simulink library "NeuroMuscularLibrary2"  (R2019b)
settings: Solver=ode45  StartTime=0.0  StopTime=10.0  RelTol=1e-3  EnableMultiTasking=on
values from neighbouring files (symbols this model uses):
  c = 0.05    [BodyMechParams.m]
  c_jointstop = 0.3 / (pi/180)    (= 17.1887338539)    [BodyMechParams.m]
  deltaLegAngleThr = 8*pi/180    (= 0.13962634016)    [CMGParams.m]
  DeltaThRef = 2e-3    (= 0.002)    [BodyMechParams.m]
  eref = 0.04    [BodyMechParams.m]
  FmaxGLU = 1500    [BodyMechParams.m]
  footBallToAnkleDist = 0.16    [BodyMechParams.m]
  footBallToCenterDist = footLength/2    (= 0.1)    [BodyMechParams.m]
  footBallToHeelDist = footLength    (= 0.2)    [BodyMechParams.m]
  footCenterToCGDist = 0.14 - footBallToCenterDist    (= 0.04)    [BodyMechParams.m]
  footInertia = 0.005    [BodyMechParams.m]
  footLength = 0.2    [BodyMechParams.m]
  footMass = 1.25    [BodyMechParams.m]
  FT_GLU = 47.6    [BodyMechParams.m]
  g = 9.80665    [BodyMechParams.m]
  groundTheta = [atan(diff(groundZ)./diff(groundX)), 0]    [generateGround.m]
  groundZ = groundZ * stepSize/(largestStep+eps)    [generateGround.m]
  hatHipToCenterDistLen = hatLength/2    (= 0.4)    [BodyMechParams.m]
  hatInertia = 3    [BodyMechParams.m]
  hatLeftHipToCenterDistWidth = .15    (= 0.15)    [BodyMechParams.m]
  hatLength = 0.8    [BodyMechParams.m]
  hatMass = 53.5    [BodyMechParams.m]
  hatThickness = 0.2    [BodyMechParams.m]
  hatWidth = 0.4    [BodyMechParams.m]
  K = 5    [BodyMechParams.m]
  k_gn = k_gn/2    (= 39226.6)    [BodyMechParams.m]
  k_gt = k_gt/2    (= 39226.6)    [BodyMechParams.m]
  k_pressure = hatMass * g / DeltaThRef    (= 262327.8875)    [BodyMechParams.m]
  legAngleSpeedMax = 10    [CMGParams.m]
  loptGAS = 0.05    [BodyMechParams.m]
  loptGLU = 0.11    [BodyMechParams.m]
  loptHAB = 0.09    [BodyMechParams.m]
  loptHAD = 0.10    (= 0.1)    [BodyMechParams.m]
  loptHAM = 0.10    (= 0.1)    [BodyMechParams.m]
  loptHFL = 0.11    [BodyMechParams.m]
  loptSOL = 0.04    [BodyMechParams.m]
  loptTA = 0.06    [BodyMechParams.m]
  loptVAS = 0.08    [BodyMechParams.m]
  lslackGAS = 0.40    (= 0.4)    [BodyMechParams.m]
  lslackGLU = 0.13    [BodyMechParams.m]
  lslackHAB = 0.07    [BodyMechParams.m]
  lslackHAD = 0.18    [BodyMechParams.m]
  lslackHAM = 0.31    [BodyMechParams.m]
  lslackHFL = 0.10    (= 0.1)    [BodyMechParams.m]
  lslackSOL = 0.26    [BodyMechParams.m]
  lslackTA = 0.24    [BodyMechParams.m]
  lslackVAS = 0.23    [BodyMechParams.m]
  mu_slide = 0.8    [BodyMechParams.m]
  mu_stick = 0.9    [BodyMechParams.m]
  N = 1.5    [BodyMechParams.m]    (also in cmaes.m = size(x,1); mergeCompareEnergyCosts.m = {S.name})
  phiKneeUpLimit = 5*pi/180    (= 0.0872664625997)    [BodyMechParams.m]
  phimaxGASa = 20*pi/180    (= 0.349065850399)    [BodyMechParams.m]
  phimaxGASk = 40*pi/180    (= 0.698131700798)    [BodyMechParams.m]
  phimaxHAMk = 0*pi/180    (= 0)    [BodyMechParams.m]
  phimaxSOL = 20*pi/180    (= 0.349065850399)    [BodyMechParams.m]
  phimaxTA = -10*pi/180    (= -0.174532925199)    [BodyMechParams.m]
  phimaxVAS = 15*pi/180    (= 0.261799387799)    [BodyMechParams.m]
  phirefGASa = -10*pi/180    (= -0.174532925199)    [BodyMechParams.m]
  phirefGASk = 15*pi/180    (= 0.261799387799)    [BodyMechParams.m]
  phirefGLU = -30*pi/180    (= -0.523598775598)    [BodyMechParams.m]
  phirefHAB = 10*pi/180    (= 0.174532925199)    [BodyMechParams.m]
  phirefHAD = 15*pi/180    (= 0.261799387799)    [BodyMechParams.m]
  phirefHAMh = -25*pi/180    (= -0.436332312999)    [BodyMechParams.m]
  phirefHAMk = 0*pi/180    (= 0)    [BodyMechParams.m]
  phirefHFL = 0*pi/180    (= 0)    [BodyMechParams.m]
  phirefSOL = -10*pi/180    (= -0.174532925199)    [BodyMechParams.m]
  phirefTA = 20*pi/180    (= 0.349065850399)    [BodyMechParams.m]
  phirefVAS = 55*pi/180    (= 0.959931088597)    [BodyMechParams.m]
  rGASa = 0.05    [BodyMechParams.m]
  rGASk = 0.05    [BodyMechParams.m]
  rGLU = 0.10    (= 0.1)    [BodyMechParams.m]
  rHAB = 0.06    [BodyMechParams.m]
  rHAD = 0.03    [BodyMechParams.m]
  rHAMh = 0.08    [BodyMechParams.m]
  rHAMk = 0.05    [BodyMechParams.m]
  rHFL = 0.10    (= 0.1)    [BodyMechParams.m]
  rhoGASa = 0.7    [BodyMechParams.m]
  rhoGASk = 0.7    [BodyMechParams.m]
  rhoGLU = 0.5    [BodyMechParams.m]
  rhoHAB = 0.7    [BodyMechParams.m]
  rhoHAD = 1    [BodyMechParams.m]
  rhoHAMh = 0.7    [BodyMechParams.m]
  rhoHAMk = 0.7    [BodyMechParams.m]
  rhoHFL = 0.5    [BodyMechParams.m]
  rhoSOL = 0.5    [BodyMechParams.m]
  rhoTA = 0.7    [BodyMechParams.m]
  rhoVAS = 0.7    [BodyMechParams.m]
  RkneeExtendGain = 25000    [CMGParams.m]
  RkneeStopGain = 12000    [CMGParams.m]
  RlegAngleFilter = 100    [CMGParams.m]
  rSOL = 0.05    [BodyMechParams.m]
  rTA = 0.04    [BodyMechParams.m]
  rVAS = 0.06    [BodyMechParams.m]
  s = x(1:N-1,:).^2 + x(2:N,:).^2    [cmaes.m]
  shankAnkleToCenterDist = shankLength/2    (= 0.25)    [BodyMechParams.m]
  shankAnkleToKneeDist = shankLength    (= 0.5)    [BodyMechParams.m]
  shankCenterToCGDist = 0.3 - shankAnkleToCenterDist    (= 0.05)    [BodyMechParams.m]
  shankInertia = 0.05    [BodyMechParams.m]
  shankLength = 0.5    [BodyMechParams.m]
  shankMass = 3.5    [BodyMechParams.m]
  tau = 0.01    [BodyMechParams.m]
  thighCenterToCGDist = 0.3 - thighKneeToCenterDist    (= 0.05)    [BodyMechParams.m]
  thighInertia = 0.15    [BodyMechParams.m]
  thighKneeToCenterDist = thighLength/2    (= 0.25)    [BodyMechParams.m]
  thighKneeToHipDist = thighLength    (= 0.5)    [BodyMechParams.m]
  thighLength = 0.5    [BodyMechParams.m]
  thighMass = 8.5    [BodyMechParams.m]
  v_gn_max = v_gz_max    (= 0.03)    [BodyMechParams.m]
  v_gt_max = v_gz_max    (= 0.03)    [BodyMechParams.m]
  v_max_pressure = 0.5    [BodyMechParams.m]
  vLimit = 0.01    [BodyMechParams.m]
  w = 0.56    [BodyMechParams.m]    (also in MuscleEnergyTest.m = 1.039; cmaes.m = ones(size(x,1)))
  w_max_jointstop = 1 * pi/180    (= 0.0174532925199)    [BodyMechParams.m]
  X = contains(N,'compareEnergyCost') .* ~contains(N,'total') .* ~contains(N,'Total')    [mergeCompareEnergyCosts.m]
undefined symbols (not defined in the file or in its folder): abdHATRef, ankleBackDriveGain, ankleCJointstop, ankleDgain, ankleFilterPID, ankleFilterSEA, ankleGearEff, ankleGearRatio, ankleIgain, ankleInitialAngle, ankleInputMass, ankleIntCoulomb, ankleIntDamping, ankleIntStatic, ankleParallelSpringDamping, ankleParallelSpringOffset, ankleParallelSpringStiffness, anklePgain, anklePlantarLimit, ankleSEADamping, ankleSEAStiffness, ankleTendonMass, ankleWMaxJointstop, dryFrictionDamping, dryFrictionStiffness, dryFrictionVelThresh, footMassp, FourBarL1, FourBarL3, GainCHAB, GainCHAD, GainGAS, GainGLU, GainHAM, GainKneeOverExt, GainSOL, GainSOLTA, GainTA, GainVAS, hipDGain, hipDGainAbd, hipPGain, hipPGainAbd, Kglu, kneeAngleOffset, kneeBackDriveGain, kneeCJointstop, kneeDgain, kneeExtCoulomb, kneeExtDamping, kneeExtendGain, kneeExtStatic, kneeFilterPID, kneeFilterSEA, kneeFlexGain, kneeGearEff, kneeGearRatio, kneeHoldGain1, kneeHoldGain2, kneeIgain ... (+62)
libraries: sm_lib x105, nesl_utility x55, simulink x22, dspswit3 x15, $bdroot x12, simulink_extras x2
(part 2 of 6)

== system NeuroMuscularLibrary2/HAT3D ==
  HAT CG : sm_lib/Frames and Transforms/Reference Frame
  HAT Center to CG : sm_lib/Frames and Transforms/Rigid Transform  TranslationMethod=Cartesian  TranslationStandardOffset=0  TranslationLengthUnit=m  TranslationStandardAxis=+Z  TranslationCartesianOffset=[0, 0, 0]  TranslationROffset=0  TranslationROffsetUnits=m  TranslationZOffset=0  TranslationZOffsetUnits=m  TranslationThetaOffset=0  TranslationThetaOffsetUnits=deg  RotationMethod=None  RotationAngleUnits=deg  RotationStandardAxis=+Z  RotationAngle=0  RotationArbitraryAxis=[0 0 1]  FollAlignAxisA=+X  BaseAlignAxisA=+Y  FollAlignAxisB=+Y  BaseAlignAxisB=+Z  RotationSequenceAxes=FollowerAxes  RotationSequence=XYX  RotationSequenceAngles=[0 0 0]  RotationSequenceAnglesUnits=deg  RotationMatrix=[1 0 0; 0 1 0; 0 0 1]
  HAT Center to Top : sm_lib/Frames and Transforms/Rigid Transform  TranslationMethod=StandardAxis  TranslationStandardOffset=hatLength/2  TranslationLengthUnit=m  TranslationStandardAxis=+Y  TranslationCartesianOffset=[0, 0, 0]  TranslationROffset=0  TranslationROffsetUnits=m  TranslationZOffset=0  TranslationZOffsetUnits=m  TranslationThetaOffset=0  TranslationThetaOffsetUnits=deg  RotationMethod=None  RotationAngleUnits=deg  RotationStandardAxis=+Z  RotationAngle=0  RotationArbitraryAxis=[0 0 1]  FollAlignAxisA=+X  BaseAlignAxisA=+Y  FollAlignAxisB=+Y  BaseAlignAxisB=+Z  RotationSequenceAxes=FollowerAxes  RotationSequence=XYX  RotationSequenceAngles=[0 0 0]  RotationSequenceAnglesUnits=deg  RotationMatrix=[1 0 0; 0 1 0; 0 0 1]
  Hip Solid : sm_lib/Body Elements/Brick Solid  GraphicAmbientColor=[0.15 0.15 0.15 1.0]  BasedOnType=Density  BrickDimensions=[hatThickness, hatLength, hatWidth]  BrickDimensionUnits=m  CenterOfMass=[0, 0, 0]  CenterOfMassUnits=m  GraphicDiffuseColor=[0.5 0.5 0.5]  Density=1000  DensityUnits=kg/(m^3)  DoExposeReferenceFrame=on  GraphicEmissiveColor=[0.0 0.0 0.0 1.0]  ExportEntireGeometry=off  SerializedFrames=<Frames/>  MarkerShape=Sphere  MarkerSize=10  GraphicType=FromGeometry  InertiaType=Custom  Mass=hatMass  MassUnits=kg  MomentsOfInertia=[0 0 hatInertia]  MomentsOfInertiaUnits=kg*m^2  GraphicOpacity=1.0  ProductsOfInertia=[0 0 0]  ProductsOfInertiaUnits=kg*m^2  GraphicShininess=75  GraphicSpecularColor=[0.5 0.5 0.5 1.0]  GraphicVisPropType=SimpleVisualProperties
  Left Hip to Center : sm_lib/Frames and Transforms/Rigid Transform  TranslationMethod=Cartesian  TranslationStandardOffset=0  TranslationLengthUnit=m  TranslationStandardAxis=+Z  TranslationCartesianOffset=[0, hatHipToCenterDistLen, hatLeftHipToCenterDistWidth]  TranslationROffset=0  TranslationROffsetUnits=m  TranslationZOffset=0  TranslationZOffsetUnits=m  TranslationThetaOffset=0  TranslationThetaOffsetUnits=deg  RotationMethod=None  RotationAngleUnits=deg  RotationStandardAxis=+Z  RotationAngle=0  RotationArbitraryAxis=[0 0 1]  FollAlignAxisA=+X  BaseAlignAxisA=+Y  FollAlignAxisB=+Y  BaseAlignAxisB=+Z  RotationSequenceAxes=FollowerAxes  RotationSequence=XYX  RotationSequenceAngles=[0 0 0]  RotationSequenceAnglesUnits=deg  RotationMatrix=[1 0 0; 0 1 0; 0 0 1]
  Left Hip to Right Hip : sm_lib/Frames and Transforms/Rigid Transform  TranslationMethod=Cartesian  TranslationStandardOffset=0  TranslationLengthUnit=m  TranslationStandardAxis=+Z  TranslationCartesianOffset=[0 0 2*hatLeftHipToCenterDistWidth]  TranslationROffset=0  TranslationROffsetUnits=m  TranslationZOffset=0  TranslationZOffsetUnits=m  TranslationThetaOffset=0  TranslationThetaOffsetUnits=deg  RotationMethod=None  RotationAngleUnits=deg  RotationStandardAxis=+Z  RotationAngle=0  RotationArbitraryAxis=[0 0 1]  FollAlignAxisA=+X  BaseAlignAxisA=+Y  FollAlignAxisB=+Y  BaseAlignAxisB=+Z  RotationSequenceAxes=FollowerAxes  RotationSequence=XYX  RotationSequenceAngles=[0 0 0]  RotationSequenceAnglesUnits=deg  RotationMatrix=[1 0 0; 0 1 0; 0 0 1]
  Mux : Mux  Inputs=2
  Mux1 : Mux  Inputs=2
  PS-Simulink Converter{,1..3} (4 alike) : nesl_utility/PS-Simulink Converter  PhysicalDomain=network_engine_domain  SubClassName=ps_output  LeftPortType=input  RightPortType=output  PseudoPeriodic=off  Frequencies=[]  Unit=1  AffineConversion=off
  To: X-forward Y-Lateral Z-up : sm_lib/Frames and Transforms/Rigid Transform  TranslationMethod=None  TranslationStandardOffset=0  TranslationLengthUnit=m  TranslationStandardAxis=+Z  TranslationCartesianOffset=[0, hatHipToCenterDistLen, -hatLeftHipToCenterDistWidth]  TranslationROffset=0  TranslationROffsetUnits=m  TranslationZOffset=0  TranslationZOffsetUnits=m  TranslationThetaOffset=0  TranslationThetaOffsetUnits=deg  RotationMethod=AlignedAxes  RotationAngleUnits=deg  RotationStandardAxis=+Z  RotationAngle=0  RotationArbitraryAxis=[0 0 1]  FollAlignAxisA=+X  BaseAlignAxisA=+Z  FollAlignAxisB=+Z  BaseAlignAxisB=+Y  RotationSequenceAxes=FollowerAxes  RotationSequence=XYX  RotationSequenceAngles=[0 0 0]  RotationSequenceAnglesUnits=deg  RotationMatrix=[1 0 0; 0 1 0; 0 0 1]
  To: Z-forward X-Lateral Y-up : sm_lib/Frames and Transforms/Rigid Transform  TranslationMethod=None  TranslationStandardOffset=0  TranslationLengthUnit=m  TranslationStandardAxis=+Z  TranslationCartesianOffset=[0, hatHipToCenterDistLen, -hatLeftHipToCenterDistWidth]  TranslationROffset=0  TranslationROffsetUnits=m  TranslationZOffset=0  TranslationZOffsetUnits=m  TranslationThetaOffset=0  TranslationThetaOffsetUnits=deg  RotationMethod=AlignedAxes  RotationAngleUnits=deg  RotationStandardAxis=+Z  RotationAngle=0  RotationArbitraryAxis=[0 0 1]  FollAlignAxisA=+Y  BaseAlignAxisA=+Y  FollAlignAxisB=+Z  BaseAlignAxisB=+X  RotationSequenceAxes=FollowerAxes  RotationSequence=XYX  RotationSequenceAngles=[0 0 0]  RotationSequenceAnglesUnits=deg  RotationMatrix=[1 0 0; 0 1 0; 0 0 1]
  Transform Sensor : sm_lib/Frames and Transforms/Transform Sensor  MeasurementFrame=World  SenseAngle=on  SenseAxis=off  SenseAngle1=off  SenseAngle2=off  SenseAngle3=off  SenseQ=off  SenseR=off  SenseOmegaX=off  SenseOmegaY=on  SenseOmegaZ=off  SenseOmega1=off  SenseOmega2=off  SenseOmega3=off  SenseQDot=off  SenseRDot=off  SenseAlphaX=off  SenseAlphaY=off  SenseAlphaZ=off  SenseAlpha1=off  SenseAlpha2=off  SenseAlpha3=off  SenseQDDot=off  SenseRDDot=off  SenseX=off  SenseY=off  SenseZ=off  SenseRad=off  SenseAzim=off  SenseDist=off  SenseInc=off  SenseXDot=off  SenseYDot=off  SenseZDot=off  SenseRadDot=off  SenseAzimDot=off  SenseDistDot=off  SenseIncDot=off  SenseXDDot=off  SenseYDDot=off  SenseZDDot=off  SenseRadDDot=off  SenseAzimDDot=off  SenseDistDDot=off  SenseIncDDot=off
  Transform Sensor : sm_lib/Frames and Transforms/Transform Sensor  MeasurementFrame=World  SenseAngle=on  SenseAxis=off  SenseAngle1=off  SenseAngle2=off  SenseAngle3=off  SenseQ=off  SenseR=off  SenseOmegaX=off  SenseOmegaY=on  SenseOmegaZ=off  SenseOmega1=off  SenseOmega2=off  SenseOmega3=off  SenseQDot=off  SenseRDot=off  SenseAlphaX=off  SenseAlphaY=off  SenseAlphaZ=off  SenseAlpha1=off  SenseAlpha2=off  SenseAlpha3=off  SenseQDDot=off  SenseRDDot=off  SenseX=off  SenseY=off  SenseZ=off  SenseRad=off  SenseAzim=off  SenseDist=off  SenseInc=off  SenseXDot=off  SenseYDot=off  SenseZDot=off  SenseRadDot=off  SenseAzimDot=off  SenseDistDot=off  SenseIncDot=off  SenseXDDot=off  SenseYDDot=off  SenseZDDot=off  SenseRadDDot=off  SenseAzimDDot=off  SenseDistDDot=off  SenseIncDDot=off
  World Frame : sm_lib/Frames and Transforms/World Frame
  Left Hip : PMIOPort  Side=Left
  Right Hip : PMIOPort  Port=2  Side=Left
  HATTop : PMIOPort  Port=3  Side=Right
  CG : PMIOPort  Port=4  Side=Right
  phiANDdphiHAT : Outport
  phiANDdphiHATAbd : Outport  Port=2
  wires:
  PS-Simulink Converter2/1 -> Mux1/1
  Mux1/1 -> phiANDdphiHATAbd/1
  PS-Simulink Converter3/1 -> Mux1/2
  PS-Simulink Converter/1 -> Mux/1
  PS-Simulink Converter1/1 -> Mux/2
  Mux/1 -> phiANDdphiHAT/1
  connections:
  Transform Sensor/RConn2 -- PS-Simulink Converter2/LConn1
  Transform Sensor/RConn3 -- PS-Simulink Converter3/LConn1
  To: Z-forward X-Lateral Y-up/RConn1 -- Transform Sensor/RConn1 -- To: X-forward Y-Lateral Z-up/LConn1
  Left Hip/RConn1 -- To: Z-forward X-Lateral Y-up/LConn1 -- Left Hip to Center/LConn1 -- Left Hip to Right Hip/LConn1
  Left Hip to Center/RConn1 -- HAT Center to CG/LConn1 -- Hip Solid/RConn1 -- HAT Center to Top/LConn1
  Right Hip/RConn1 -- Left Hip to Right Hip/RConn1
  World Frame/RConn1 -- Transform Sensor/LConn1
  PS-Simulink Converter/LConn1 -- Transform Sensor/RConn2
  Transform Sensor/RConn3 -- PS-Simulink Converter1/LConn1
  To: X-forward Y-Lateral Z-up/RConn1 -- Transform Sensor/RConn1
  HAT CG/RConn1 -- HAT Center to CG/RConn1 -- CG/RConn1
  HATTop/RConn1 -- HAT Center to Top/RConn1

== system NeuroMuscularLibrary2/HFL Link ==
  note: HFL Attachment
  hip angle [rad] : Inport
  Constant : Constant  Value=lslackHFL+loptHFL
  Constant1 : Constant  Value=rHFL
  Constant2 : Constant  Value=phirefHFL
  Gain2 : Gain  Gain=rhoHFL
  Product : Product  RndMeth=Zero
  Sum2 : Sum  Inputs=|+-
  Sum5 : Sum  Inputs=|++
  lmtu [m] : Outport
  lever [m] : Outport  Port=2
  wires:
  Constant/1 -> Sum5/1
  Sum5/1 -> lmtu [m]/1
  Product/1 -> Gain2/1
  hip angle [rad]/1 -> Sum2/1
  Constant2/1 -> Sum2/2
  Sum2/1 -> Product/1
  Constant1/1 -> Product/2, lever [m]/1
  Gain2/1 -> Sum5/2

== system NeuroMuscularLibrary2/Hard Stops ==
  Ideal Torques : Inport
  Muscle Torques : Inport  Port=2
  phiANDdphiHip : Inport  Port=3
  phiANDdphiKnee : Inport  Port=4
  phiANDdphiAnkle : Inport  Port=5
  Add : Sum  Inputs=+++
  Ankle Joint Limit : $bdroot/Overextension//Overflexion Joint Limit  phiUpLimit=phiAnkleUpLimit  phiLowLimit=phiAnkleLowLimit
  Demux : Demux  Outputs=2
  Demux1 : Demux  Outputs=2
  Demux2 : Demux  Outputs=2
  Hip Overextension Joint Limit : $bdroot/Overextension Joint Limit  phiUpLimit=phiHipUpLimit  ext=1
  Knee Overextension Joint Limit : $bdroot/Overextension Joint Limit  phiUpLimit=phiKneeUpLimit  ext=-1
  Mux : Mux  Inputs=3
  Over Extended Knee? : simulink/Logic and Bit Operations/Compare To Constant  relop=<  const=-5*pi/180  OutDataTypeStr=boolean
  Product1 : Product
  Net Torque : Outport
  Hip Stop Torque : Outport  Port=2
  Knee Stop Torque : Outport  Port=3
  Ankle Stop Torque : Outport  Port=4
  wires:
  Ideal Torques/1 -> Add/1
  Add/1 -> Net Torque/1
  phiANDdphiAnkle/1 -> Demux2/1
  phiANDdphiHip/1 -> Demux1/1
  Hip Overextension Joint Limit/1 -> Mux/1, Hip Stop Torque/1
  phiANDdphiKnee/1 -> Demux/1
  Demux2/2 -> Ankle Joint Limit/2
  Demux2/1 -> Ankle Joint Limit/1
  Demux1/2 -> Hip Overextension Joint Limit/2
  Demux1/1 -> Hip Overextension Joint Limit/1
  Demux/1 -> Knee Overextension Joint Limit/1, Over Extended Knee?/1
  Demux/2 -> Knee Overextension Joint Limit/2
  Over Extended Knee?/1 -> Product1/2
  Ankle Joint Limit/1 -> Mux/3, Ankle Stop Torque/1
  Mux/1 -> Add/3
  Muscle Torques/1 -> Add/2
  Knee Overextension Joint Limit/1 -> Product1/1, Mux/2
  Product1/1 -> Knee Stop Torque/1

== system NeuroMuscularLibrary2/Hard Stops 3D ==
  Ideal Torques : Inport
  Muscle Torques : Inport  Port=2
  phiANDdphiHip : Inport  Port=3
  phiANDdphiKnee : Inport  Port=4
  phiANDdphiAnkle : Inport  Port=5
  phiANDdphiHipAbd : Inport  Port=6
  Add : Sum  Inputs=+++
  Ankle Joint Limit : $bdroot/Overextension//Overflexion Joint Limit  phiUpLimit=phiAnkleUpLimit  phiLowLimit=phiAnkleLowLimit
  Demux{,1..3} (4 alike) : Demux  Outputs=2
  Hip Abduction Joint Limit : $bdroot/Overextension//Overflexion Joint Limit  phiUpLimit=phiHipAbdUpLimit  phiLowLimit=phiHipAbdLowLimit
  Hip Overextension Joint Limit : $bdroot/Overextension Joint Limit  phiUpLimit=phiHipUpLimit  ext=1
  Knee Overextension Joint Limit : $bdroot/Overextension Joint Limit  phiUpLimit=phiKneeUpLimit  ext=-1
  Mux : Mux
  Over Extended Knee? : simulink/Logic and Bit Operations/Compare To Constant  relop=<  const=-5*pi/180  OutDataTypeStr=boolean
  Product1 : Product
  Net Torque : Outport
  Hip Stop Torque : Outport  Port=2
  Knee Stop Torque : Outport  Port=3
  Ankle Stop Torque : Outport  Port=4
  Hip Abd Stop Torque : Outport  Port=5
  wires:
  Product1/1 -> Knee Stop Torque/1
  Knee Overextension Joint Limit/1 -> Mux/2, Product1/1
  Muscle Torques/1 -> Add/2
  Mux/1 -> Add/3
  Ankle Joint Limit/1 -> Ankle Stop Torque/1, Mux/3
  Over Extended Knee?/1 -> Product1/2
  Demux/2 -> Knee Overextension Joint Limit/2
  Demux/1 -> Over Extended Knee?/1, Knee Overextension Joint Limit/1
  Demux1/1 -> Hip Overextension Joint Limit/1
  Demux1/2 -> Hip Overextension Joint Limit/2
  Demux2/1 -> Ankle Joint Limit/1
  Demux2/2 -> Ankle Joint Limit/2
  phiANDdphiKnee/1 -> Demux/1
  Hip Overextension Joint Limit/1 -> Hip Stop Torque/1, Mux/1
  phiANDdphiHip/1 -> Demux1/1
  phiANDdphiAnkle/1 -> Demux2/1
  Add/1 -> Net Torque/1
  Ideal Torques/1 -> Add/1
  phiANDdphiHipAbd/1 -> Demux3/1
  Demux3/1 -> Hip Abduction Joint Limit/1
  Demux3/2 -> Hip Abduction Joint Limit/2
  Hip Abduction Joint Limit/1 -> Hip Abd Stop Torque/1, Mux/4

== system NeuroMuscularLibrary2/Hill Muscle ==
  note: Muscle-Tendon Dynamics
  note: Excitation Contraction Coupling
  STIM : Inport
  lmtc [m] : Inport  Port=2
  1 : Product  Inputs=**  SaturateOnIntegerOverflow=on  InputSameDT=on  OutDataTypeStr=Inherit: Same as first input
  1/lslack : Gain  Gain=1/lslack  SaturateOnIntegerOverflow=on  OutDataTypeStr=Inherit: Same as input  ParamDataTypeStr=Inherit: Same as input
  BE force-length relation : Subsystem
  CE force-length relation : Subsystem
  CE inverse force-velocity relation : Subsystem
  Constant : Constant  Value=lslack
  ECC TransferFcn : simulink_extras/Additional Linear/Transfer Fcn (with initial outputs)  N=[1]  D="[tau  1]"  Y0=preA  U0=0
      settings: AttributesFormatString=pre-activation: %<Y0>
  Fmax : Gain  Gain=Fmax  SaturateOnIntegerOverflow=on  OutDataTypeStr=Inherit: Same as input  ParamDataTypeStr=Inherit: Same as input
  Fv = Fse / (A*Fce) : Product  Inputs=*/  SaturateOnIntegerOverflow=on  InputSameDT=on  OutDataTypeStr=Inherit: Same as first input
  Integrator : Integrator  InitialConditionSource=external  LowerSaturationLimit=0.05
  PE force-length relation : Subsystem
  SE force-length relation : Subsystem
  Sum : Sum  Inputs=|+-  SaturateOnIntegerOverflow=on  InputSameDT=on  OutDataTypeStr=Inherit: Same as first input
  Sum2 : Sum  Inputs=|-+  SaturateOnIntegerOverflow=on  InputSameDT=on  OutDataTypeStr=Inherit: Same as first input
  Sum3 : Sum  SaturateOnIntegerOverflow=on  InputSameDT=on  OutDataTypeStr=Inherit: Same as first input
  Sum4 : Sum  SaturateOnIntegerOverflow=on  InputSameDT=on  OutDataTypeStr=Inherit: Same as first input
  lce/lopt : Gain  Gain=1/lopt  SaturateOnIntegerOverflow=on  OutDataTypeStr=Inherit: Same as input  ParamDataTypeStr=Inherit: Same as input
  vmax*lopt : Gain  Gain=vmax*lopt  SaturateOnIntegerOverflow=on  OutDataTypeStr=Inherit: Same as input  ParamDataTypeStr=Inherit: Same as input
  Fmtc : Outport  InitialOutput=0
  Lce : Outport  Port=2  InitialOutput=0
  Vce : Outport  Port=3  InitialOutput=0
  Lse : Outport  Port=4  InitialOutput=0
  A : Outport  Port=5  InitialOutput=0
  wires:
  Integrator/1 -> Sum/2, lce/lopt/1, Lce/1  "lce"
  Sum/1 -> 1/lslack/1, Lse/1  "lse"
  lce/lopt/1 -> CE force-length relation/1(lce [lopt]), BE force-length relation/1(lce [lopt]), PE force-length relation/1(lce [lopt])
  Fv = Fse / (A*Fce)/1 -> CE inverse force-velocity relation/1(Fv[Fmax])  "fv"
  vmax*lopt/1 -> Integrator/1, Vce/1  "vce"
  lmtc [m]/1 -> Sum2/2, Sum/1  "lmtc"
  Fmax/1 -> Fmtc/1  "Fmtc"
  1/lslack/1 -> SE force-length relation/1(lse [lslack])
  SE force-length relation/1(fse [Fmax]) -> Fmax/1, Sum4/1
  Sum2/1 -> Integrator/2
  Constant/1 -> Sum2/1
  CE force-length relation/1(fce [Fmax]) -> 1/1
  Sum4/1 -> Fv = Fse / (A*Fce)/1
  PE force-length relation/1(fpe [Fmax]) -> Sum3/1
  1/1 -> Sum3/2
  BE force-length relation/1(fbe [Fmax]) -> Sum4/2
  Sum3/1 -> Fv = Fse / (A*Fce)/2
  CE inverse force-velocity relation/1(v[vmax]) -> vmax*lopt/1
  STIM/1 -> ECC TransferFcn/1
  ECC TransferFcn/1 -> A/1, 1/2

== system NeuroMuscularLibrary2/Leg Angle//Length ==
  Constant : Constant  Value=pi
  Demux : Demux  Outputs=2
  Mux : Mux  Inputs=3
  Mux1 : Mux  Inputs=3
  PS-Simulink Converter{,1..6} (7 alike) : nesl_utility/PS-Simulink Converter  PhysicalDomain=network_engine_domain  SubClassName=ps_output  LeftPortType=input  RightPortType=output  PseudoPeriodic=off  Frequencies=[]  Unit=m  AffineConversion=off
  Position Sensor : sm_lib/Frames and Transforms/Transform Sensor  MeasurementFrame=World  SenseAngle=off  SenseAxis=off  SenseAngle1=off  SenseAngle2=off  SenseAngle3=off  SenseQ=off  SenseR=off  SenseOmegaX=off  SenseOmegaY=off  SenseOmegaZ=off  SenseOmega1=off  SenseOmega2=off  SenseOmega3=off  SenseQDot=off  SenseRDot=off  SenseAlphaX=off  SenseAlphaY=off  SenseAlphaZ=off  SenseAlpha1=off  SenseAlpha2=off  SenseAlpha3=off  SenseQDDot=off  SenseRDDot=off  SenseX=on  SenseY=on  SenseZ=on  SenseRad=off  SenseAzim=off  SenseDist=off  SenseInc=off  SenseXDot=off  SenseYDot=off  SenseZDot=off  SenseRadDot=off  SenseAzimDot=off  SenseDistDot=off  SenseIncDot=off  SenseXDDot=off  SenseYDDot=off  SenseZDDot=off  SenseRadDDot=off  SenseAzimDDot=off  SenseDistDDot=off  SenseIncDDot=off
  Position Sensor1 : sm_lib/Frames and Transforms/Transform Sensor  MeasurementFrame=World  SenseAngle=off  SenseAxis=off  SenseAngle1=off  SenseAngle2=off  SenseAngle3=off  SenseQ=off  SenseR=off  SenseOmegaX=off  SenseOmegaY=off  SenseOmegaZ=off  SenseOmega1=off  SenseOmega2=off  SenseOmega3=off  SenseQDot=off  SenseRDot=off  SenseAlphaX=off  SenseAlphaY=off  SenseAlphaZ=off  SenseAlpha1=off  SenseAlpha2=off  SenseAlpha3=off  SenseQDDot=off  SenseRDDot=off  SenseX=on  SenseY=on  SenseZ=on  SenseRad=off  SenseAzim=off  SenseDist=off  SenseInc=off  SenseXDot=off  SenseYDot=off  SenseZDot=off  SenseRadDot=off  SenseAzimDot=off  SenseDistDot=off  SenseIncDot=off  SenseXDDot=off  SenseYDDot=off  SenseZDDot=off  SenseRadDDot=off  SenseAzimDDot=off  SenseDistDDot=off  SenseIncDDot=off
  Selector : Selector  InputPortWidth=3  IndexOptions=Index vector (dialog)  Indices=[3 1]  OutputSizes=1
  Subtract : Sum  Inputs=+-
  Sum : Sum  Inputs=|-+
  Transform Sensor : sm_lib/Frames and Transforms/Transform Sensor  MeasurementFrame=World  SenseAngle=off  SenseAxis=off  SenseAngle1=off  SenseAngle2=off  SenseAngle3=off  SenseQ=off  SenseR=off  SenseOmegaX=off  SenseOmegaY=off  SenseOmegaZ=off  SenseOmega1=off  SenseOmega2=off  SenseOmega3=off  SenseQDot=off  SenseRDot=off  SenseAlphaX=off  SenseAlphaY=off  SenseAlphaZ=off  SenseAlpha1=off  SenseAlpha2=off  SenseAlpha3=off  SenseQDDot=off  SenseRDDot=off  SenseX=off  SenseY=off  SenseZ=off  SenseRad=off  SenseAzim=off  SenseDist=on  SenseInc=off  SenseXDot=off  SenseYDot=off  SenseZDot=off  SenseRadDot=off  SenseAzimDot=off  SenseDistDot=off  SenseIncDot=off  SenseXDDot=off  SenseYDDot=off  SenseZDDot=off  SenseRadDDot=off  SenseAzimDDot=off  SenseDistDDot=off  SenseIncDDot=off
  Trigonometric Function : Trigonometry  Operator=atan2  OutputSignalType=real
  World Frame : sm_lib/Frames and Transforms/World Frame
  Hip : PMIOPort  Side=Left
  Ankle : PMIOPort  Port=2  Side=Left
  Leg Angle : Outport
  Leg Length : Outport  Port=2
  wires:
  PS-Simulink Converter6/1 -> Leg Length/1
  PS-Simulink Converter2/1 -> Mux/3
  PS-Simulink Converter/1 -> Mux/1
  PS-Simulink Converter1/1 -> Mux/2
  PS-Simulink Converter5/1 -> Mux1/3
  PS-Simulink Converter3/1 -> Mux1/1
  PS-Simulink Converter4/1 -> Mux1/2
  Mux/1 -> Subtract/1
  Mux1/1 -> Subtract/2
  Trigonometric Function/1 -> Sum/1
  Sum/1 -> Leg Angle/1  "Saggital leg angle"
  Constant/1 -> Sum/2
  Subtract/1 -> Selector/1
  Selector/1 -> Demux/1
  Demux/1 -> Trigonometric Function/1
  Demux/2 -> Trigonometric Function/2
  connections:
  PS-Simulink Converter6/LConn1 -- Transform Sensor/RConn2
  PS-Simulink Converter2/LConn1 -- Position Sensor/RConn4
  PS-Simulink Converter/LConn1 -- Position Sensor/RConn2
  Transform Sensor/RConn1 -- Hip/RConn1 -- Position Sensor/RConn1
  PS-Simulink Converter1/LConn1 -- Position Sensor/RConn3
  World Frame/RConn1 -- Position Sensor/LConn1 -- Position Sensor1/LConn1
  PS-Simulink Converter4/LConn1 -- Position Sensor1/RConn3
  PS-Simulink Converter5/LConn1 -- Position Sensor1/RConn4
  PS-Simulink Converter3/LConn1 -- Position Sensor1/RConn2
  Transform Sensor/LConn1 -- Ankle/RConn1 -- Position Sensor1/RConn1

== system NeuroMuscularLibrary2/Leg Angle//Length3D ==
  Constant : Constant  Value=pi
  Constant1 : Constant  Value=0
  Demux : Demux  Outputs=2
  Demux1 : Demux  Outputs=2
  Mux : Mux  Inputs=3
  Mux1 : Mux  Inputs=3
  Mux2 : Mux  Inputs=2
  PS-Simulink Converter{,1..6} (7 alike) : nesl_utility/PS-Simulink Converter  PhysicalDomain=network_engine_domain  SubClassName=ps_output  LeftPortType=input  RightPortType=output  PseudoPeriodic=off  Frequencies=[]  Unit=m  AffineConversion=off
  Position Sensor : sm_lib/Frames and Transforms/Transform Sensor  MeasurementFrame=World  SenseAngle=off  SenseAxis=off  SenseAngle1=off  SenseAngle2=off  SenseAngle3=off  SenseQ=off  SenseR=off  SenseOmegaX=off  SenseOmegaY=off  SenseOmegaZ=off  SenseOmega1=off  SenseOmega2=off  SenseOmega3=off  SenseQDot=off  SenseRDot=off  SenseAlphaX=off  SenseAlphaY=off  SenseAlphaZ=off  SenseAlpha1=off  SenseAlpha2=off  SenseAlpha3=off  SenseQDDot=off  SenseRDDot=off  SenseX=on  SenseY=on  SenseZ=on  SenseRad=off  SenseAzim=off  SenseDist=off  SenseInc=off  SenseXDot=off  SenseYDot=off  SenseZDot=off  SenseRadDot=off  SenseAzimDot=off  SenseDistDot=off  SenseIncDot=off  SenseXDDot=off  SenseYDDot=off  SenseZDDot=off  SenseRadDDot=off  SenseAzimDDot=off  SenseDistDDot=off  SenseIncDDot=off
  Position Sensor1 : sm_lib/Frames and Transforms/Transform Sensor  MeasurementFrame=World  SenseAngle=off  SenseAxis=off  SenseAngle1=off  SenseAngle2=off  SenseAngle3=off  SenseQ=off  SenseR=off  SenseOmegaX=off  SenseOmegaY=off  SenseOmegaZ=off  SenseOmega1=off  SenseOmega2=off  SenseOmega3=off  SenseQDot=off  SenseRDot=off  SenseAlphaX=off  SenseAlphaY=off  SenseAlphaZ=off  SenseAlpha1=off  SenseAlpha2=off  SenseAlpha3=off  SenseQDDot=off  SenseRDDot=off  SenseX=on  SenseY=on  SenseZ=on  SenseRad=off  SenseAzim=off  SenseDist=off  SenseInc=off  SenseXDot=off  SenseYDot=off  SenseZDot=off  SenseRadDot=off  SenseAzimDot=off  SenseDistDot=off  SenseIncDot=off  SenseXDDot=off  SenseYDDot=off  SenseZDDot=off  SenseRadDDot=off  SenseAzimDDot=off  SenseDistDDot=off  SenseIncDDot=off
  Selector : Selector  InputPortWidth=3  IndexOptions=Index vector (dialog)  Indices=[3 1]  OutputSizes=1
  Selector1 : Selector  InputPortWidth=3  IndexOptions=Index vector (dialog)  Indices=[3 2]  OutputSizes=1
  Subtract : Sum  Inputs=+-
  Sum : Sum  Inputs=|-+
  Sum1 : Sum  Inputs=|++
  Transform Sensor : sm_lib/Frames and Transforms/Transform Sensor  MeasurementFrame=World  SenseAngle=off  SenseAxis=off  SenseAngle1=off  SenseAngle2=off  SenseAngle3=off  SenseQ=off  SenseR=off  SenseOmegaX=off  SenseOmegaY=off  SenseOmegaZ=off  SenseOmega1=off  SenseOmega2=off  SenseOmega3=off  SenseQDot=off  SenseRDot=off  SenseAlphaX=off  SenseAlphaY=off  SenseAlphaZ=off  SenseAlpha1=off  SenseAlpha2=off  SenseAlpha3=off  SenseQDDot=off  SenseRDDot=off  SenseX=off  SenseY=off  SenseZ=off  SenseRad=off  SenseAzim=off  SenseDist=on  SenseInc=off  SenseXDot=off  SenseYDot=off  SenseZDot=off  SenseRadDot=off  SenseAzimDot=off  SenseDistDot=off  SenseIncDot=off  SenseXDDot=off  SenseYDDot=off  SenseZDDot=off  SenseRadDDot=off  SenseAzimDDot=off  SenseDistDDot=off  SenseIncDDot=off
  Trigonometric Function : Trigonometry  Operator=atan2  OutputSignalType=real
  Trigonometric Function1 : Trigonometry  Operator=atan2  OutputSignalType=real
  World Frame : sm_lib/Frames and Transforms/World Frame
  Hip : PMIOPort  Side=Left
  Ankle : PMIOPort  Port=2  Side=Left
  Leg Angle : Outport
  Leg Length : Outport  Port=2
  wires:
  Sum1/1 -> Mux2/2  "Coronal leg angle"
  Trigonometric Function1/1 -> Sum1/1
  Constant1/1 -> Sum1/2
  Demux1/2 -> Trigonometric Function1/2
  Selector1/1 -> Demux1/1
  Demux1/1 -> Trigonometric Function1/1
  Mux2/1 -> Leg Angle/1
  Demux/2 -> Trigonometric Function/2
  Demux/1 -> Trigonometric Function/1
  Selector/1 -> Demux/1
  Subtract/1 -> Selector/1, Selector1/1
  Constant/1 -> Sum/2
  Sum/1 -> Mux2/1  "Saggital leg angle"
  Trigonometric Function/1 -> Sum/1
  Mux1/1 -> Subtract/2
  Mux/1 -> Subtract/1
  PS-Simulink Converter4/1 -> Mux1/2
  PS-Simulink Converter3/1 -> Mux1/1
  PS-Simulink Converter5/1 -> Mux1/3
  PS-Simulink Converter1/1 -> Mux/2
  PS-Simulink Converter/1 -> Mux/1
  PS-Simulink Converter2/1 -> Mux/3
  PS-Simulink Converter6/1 -> Leg Length/1
  connections:
  Position Sensor1/RConn1 -- Ankle/RConn1 -- Transform Sensor/LConn1
  PS-Simulink Converter3/LConn1 -- Position Sensor1/RConn2
  PS-Simulink Converter5/LConn1 -- Position Sensor1/RConn4
  PS-Simulink Converter4/LConn1 -- Position Sensor1/RConn3
  Position Sensor1/LConn1 -- Position Sensor/LConn1 -- World Frame/RConn1
  PS-Simulink Converter1/LConn1 -- Position Sensor/RConn3
  Position Sensor/RConn1 -- Hip/RConn1 -- Transform Sensor/RConn1
  PS-Simulink Converter/LConn1 -- Position Sensor/RConn2
  PS-Simulink Converter2/LConn1 -- Position Sensor/RConn4
  PS-Simulink Converter6/LConn1 -- Transform Sensor/RConn2

== system NeuroMuscularLibrary2/Lower Thigh ==
  Knee Solid : sm_lib/Body Elements/Cylindrical Solid  GraphicAmbientColor=[0.15 0.15 0.15 1.0]  BasedOnType=Density  CenterOfMass=[0 0 thighCenterToCGDist*ThPos]  CenterOfMassUnits=m  GraphicDiffuseColor=[0.5 0.5 0.5]  CylinderLength=thighLength*ThPos  CylinderLengthUnits=m  CylinderRadius=.075  CylinderRadiusUnits=m  Density=1000  DensityUnits=kg/(m^3)  DoExposeReferenceFrame=on  GraphicEmissiveColor=[0.0 0.0 0.0 1.0]  ExportEntireGeometry=off  SerializedFrames=<Frames/>  MarkerShape=Sphere  MarkerSize=10  GraphicType=FromGeometry  InertiaType=Custom  Mass=thighMass*ThPos  MassUnits=kg  MomentsOfInertia=[thighInertia*(ThPos)^3 0 0]  MomentsOfInertiaUnits=kg*m^2  GraphicOpacity=1.0  ProductsOfInertia=[0 0 0]  ProductsOfInertiaUnits=kg*m^2  GraphicShininess=75  GraphicSpecularColor=[0.5 0.5 0.5 1.0]  GraphicVisPropType=SimpleVisualProperties
  Knee to Center : sm_lib/Frames and Transforms/Rigid Transform  TranslationMethod=Cartesian  TranslationStandardOffset=0  TranslationLengthUnit=m  TranslationStandardAxis=+Z  TranslationCartesianOffset=[0 thighKneeToCenterDist*ThPos 0]  TranslationROffset=0  TranslationROffsetUnits=m  TranslationZOffset=0  TranslationZOffsetUnits=m  TranslationThetaOffset=0  TranslationThetaOffsetUnits=deg  RotationMethod=AlignedAxes  RotationAngleUnits=deg  RotationStandardAxis=+Z  RotationAngle=0  RotationArbitraryAxis=[0 0 1]  FollAlignAxisA=+Z  BaseAlignAxisA=+Y  FollAlignAxisB=+X  BaseAlignAxisB=+X  RotationSequenceAxes=FollowerAxes  RotationSequence=XYX  RotationSequenceAngles=[0 0 0]  RotationSequenceAnglesUnits=deg  RotationMatrix=[1 0 0; 0 1 0; 0 0 1]
  Knee to Sensor Sheet : sm_lib/Frames and Transforms/Rigid Transform  TranslationMethod=Cartesian  TranslationStandardOffset=0  TranslationLengthUnit=m  TranslationStandardAxis=+Z  TranslationCartesianOffset=[0 thighKneeToHipDist*ThPos 0]  TranslationROffset=0  TranslationROffsetUnits=m  TranslationZOffset=0  TranslationZOffsetUnits=m  TranslationThetaOffset=0  TranslationThetaOffsetUnits=deg  RotationMethod=None  RotationAngleUnits=deg  RotationStandardAxis=+Z  RotationAngle=0  RotationArbitraryAxis=[0 0 1]  FollAlignAxisA=+Z  BaseAlignAxisA=+X  FollAlignAxisB=+Y  BaseAlignAxisB=+Y  RotationSequenceAxes=FollowerAxes  RotationSequence=XYX  RotationSequenceAngles=[0 0 0]  RotationSequenceAnglesUnits=deg  RotationMatrix=[1 0 0; 0 1 0; 0 0 1]
  Thigh CG : sm_lib/Frames and Transforms/Reference Frame
  Thigh Center to CG : sm_lib/Frames and Transforms/Rigid Transform  TranslationMethod=Cartesian  TranslationStandardOffset=0  TranslationLengthUnit=m  TranslationStandardAxis=+Z  TranslationCartesianOffset=[0 0 thighCenterToCGDist*ThPos]  TranslationROffset=0  TranslationROffsetUnits=m  TranslationZOffset=0  TranslationZOffsetUnits=m  TranslationThetaOffset=0  TranslationThetaOffsetUnits=deg  RotationMethod=None  RotationAngleUnits=deg  RotationStandardAxis=+Z  RotationAngle=0  RotationArbitraryAxis=[0 0 1]  FollAlignAxisA=+X  BaseAlignAxisA=+Y  FollAlignAxisB=+Y  BaseAlignAxisB=+Z  RotationSequenceAxes=FollowerAxes  RotationSequence=XYX  RotationSequenceAngles=[0 0 0]  RotationSequenceAnglesUnits=deg  RotationMatrix=[1 0 0; 0 1 0; 0 0 1]
  Knee : PMIOPort  Side=Left
  Sensor Sheet : PMIOPort  Port=2  Side=Right
  connections:
  Knee/RConn1 -- Knee to Center/LConn1 -- Knee to Sensor Sheet/LConn1
  Knee to Center/RConn1 -- Knee Solid/RConn1 -- Thigh Center to CG/LConn1
  Knee to Sensor Sheet/RConn1 -- Sensor Sheet/RConn1
  Thigh Center to CG/RConn1 -- Thigh CG/RConn1

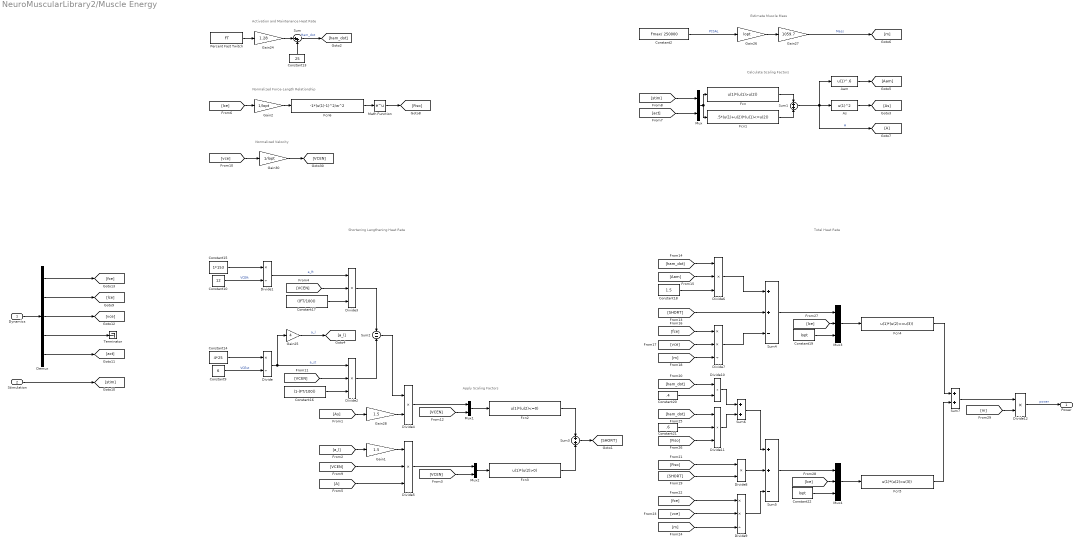
== system NeuroMuscularLibrary2/Muscle Energy ==
  note: Total Heat Rate
  note: Estimate Muscle Mass
  note: Calculate Scaling Factors
  note: Apply Scaling Factors
  note: Shortening Lengthening Heat Rate
  note: Normalized Velocity
  note: Normalized Force-Length Relationship
  note: Activation and Maintenance Heat Rate
  Dynamics : Inport
  Stimulation : Inport  Port=2
  "Aam " : Fcn  Expr=u(1)^.6
  As : Fcn  Expr=u(1)^2
  Constant10 : Constant  Value=12
  Constant13 : Constant  Value=25
  Constant14 : Constant  Value=4*25
  Constant15 : Constant  Value=1*153
  Constant16 : Constant  Value=(1-(FT/100))
  Constant17 : Constant  Value=((FT/100))
  Constant18 : Constant  Value=1.5
  Constant19 : Constant  Value=lopt
  Constant2 : Constant  Value=Fmax/ 250000
  Constant20 : Constant  Value=.4
  Constant21 : Constant  Value=.6
  Constant22 : Constant  Value=lopt
  Constant9 : Constant  Value=6
  Demux : Demux  Outputs=5
  Divide : Product  Inputs=*/
  Divide1 : Product  Inputs=*/
  Divide{4,8,10,12} (4 alike) : Product  Inputs=**
  Divide{2..3,5..6,11} (5 alike) : Product  Inputs=***
  Divide7 : Product  Inputs=**/
  Divide9 : Product  Inputs=**/
  Fcn : Fcn  Expr=u(1)*(u(1)>u(2))
  Fcn1 : Fcn  Expr=.5*(u(1)+u(2))*(u(1)<=u(2))
  Fcn2 : Fcn  Expr=u(1)*(u(2)<=0)
  Fcn3 : Fcn  Expr=u(1)*(u(2)>0)
  Fcn4 : Fcn  Expr=u(1)*(u(2)<=u(3))
  Fcn5 : Fcn  Expr=u(1)*(u(2)>u(3))
  Fcn6 : Fcn  Expr=-1*(u(1)-1)^2/w^2
  Gain1 : Gain  Gain=1.5
  Gain2 : Gain  Gain=1/lopt
  Gain24 : Gain  Gain=1.28
  Gain25 : Gain  Gain=4
  Gain26 : Gain  Gain=lopt
  Gain27 : Gain  Gain=1059.7
  Gain28 : Gain  Gain=1.5
  Gain30 : Gain  Gain=1/lopt
  Math Function : Math  SaturateOnIntegerOverflow=on
  Mux : Mux  Inputs=2
  Mux1 : Mux  Inputs=2
  Mux2 : Mux  Inputs=2
  Mux3 : Mux  Inputs=3
  Mux4 : Mux  Inputs=3
  Percent Fast Twitch : Constant  Value=FT
  Sum : Sum  Inputs=|++
  Sum1 : Sum  Inputs=+|+
  Sum2 : Sum  Inputs=-|-
  Sum3 : Sum  Inputs=+|+
  Sum4 : Sum  Inputs=++-
  Sum5 : Sum  Inputs=++-
  Sum6 : Sum
  Sum7 : Sum
  Terminator : Terminator
  Power : Outport
  wires:
  Gain2/1 -> Fcn6/1
  [lce] -> Gain2/1
  Demux/4 -> Terminator/1
  Demux/5 -> [act]
  Demux/3 -> [vce]
  Demux/2 -> [lce]
  Demux/1 -> [fce]
  Stimulation/1 -> [stim]
  Dynamics/1 -> Demux/1
  [As] -> Gain28/1
  Fcn2/1 -> Sum3/1
  Sum3/1 -> [SHORT]
  Mux2/1 -> Fcn3/1
  Gain30/1 -> [VCEN]
  Gain27/1 -> [m]  "Mass"
  Constant9/1 -> Divide/2  "VCEst"
  Gain28/1 -> Divide4/2
  [lce] -> Mux3/2
  Mux3/1 -> Fcn4/1
  [SHORT] -> Divide8/2
  Constant2/1 -> Gain26/1  "PCSAL"
  Constant21/1 -> Divide11/2
  [VCEN] -> Mux2/2
  Percent Fast Twitch/1 -> Gain24/1
  Mux/1 -> Fcn/1, Fcn1/1
  Sum/1 -> [ham_dot]  "Ham_dot"
  [fce] -> Divide9/1
  [m] -> Divide7/3
  Sum2/1 -> Divide4/1
  Constant20/1 -> Divide10/2
  As/1 -> [As]
  Divide8/1 -> Sum5/2
  Constant13/1 -> Sum/2
  Divide7/1 -> Sum4/3
  [vce] -> Divide9/2
  Fcn/1 -> Sum1/1
  Fcn1/1 -> Sum1/2
  [VCEN] -> Divide3/2
  Mux1/1 -> Fcn2/1
  Divide4/1 -> Mux1/1
  Constant15/1 -> Divide1/1
  Constant18/1 -> Divide6/3
  Sum1/1 -> [A], As/1, "Aam "/1  "A"
  [ham_dot] -> Divide6/1
  Divide/1 -> Divide2/1, Gain25/1  "a_st"
  Divide6/1 -> Sum4/1
  Constant14/1 -> Divide/1
  Divide5/1 -> Mux2/1
  Constant22/1 -> Mux4/3
  Fcn3/1 -> Sum3/2
  Sum7/1 -> Divide12/1
  [VCEN] -> Mux1/2
  Divide1/1 -> Divide3/1  "a_ft"
  [VCEN] -> Divide2/2
  Divide2/1 -> Sum2/2
  Constant10/1 -> Divide1/2  "VCEft"
  "Aam "/1 -> [Aam]
  Math Function/1 -> [Fiso]
  Gain25/1 -> [a_l]  "a_l"
  Divide3/1 -> Sum2/1
  [vce] -> Divide7/2
  [Fiso] -> Divide11/3
  Constant17/1 -> Divide3/3
  Constant16/1 -> Divide2/3
  Gain1/1 -> Divide5/1
  [Aam] -> Divide6/2
  [a_l] -> Gain1/1
  [VCEN] -> Divide5/2
  Fcn5/1 -> Sum7/2
  Mux4/1 -> Fcn5/1
  Constant19/1 -> Mux3/3
  [SHORT] -> Sum4/2
  Sum6/1 -> Sum5/1
  Sum5/1 -> Mux4/1
  [ham_dot] -> Divide10/1
  [lce] -> Mux4/2
  [m] -> Divide9/3
  Divide11/1 -> Sum6/2
  [ham_dot] -> Divide11/1
  [A] -> Divide5/3
  Fcn6/1 -> Math Function/1
  [Fiso] -> Divide8/1
  Fcn4/1 -> Sum7/1
  Divide12/1 -> Power/1  "power"
  Sum4/1 -> Mux3/1
  Divide9/1 -> Sum5/3
  Divide10/1 -> Sum6/1
  Gain24/1 -> Sum/1
  Gain26/1 -> Gain27/1
  [stim] -> Mux/1
  [act] -> Mux/2
  [vce] -> Gain30/1
  [fce] -> Divide7/1
  [m] -> Divide12/2

== system NeuroMuscularLibrary2/Overextension Joint Limit ==
  note: Knee/Hip Joint Limits
  phi [rad] : Inport
  dphi [rad/s] : Inport  Port=2
  Gain1 : Gain  Gain=ext
  Gain2 : Gain  Gain=-ext
  Gain3 : Gain  Gain=c_jointstop
  Gain4 : Gain  Gain=1/w_max_jointstop
  Gain5 : Gain  Gain=ext
  Limit Ankle Range : simulink/Logic and Bit Operations/Interval Test  Commented=on  IntervalClosedRight=on  uplimit=185*pi/180  IntervalClosedLeft=on  lowlimit=40*pi/180  OutDataTypeStr=boolean
  Logical Operator3 : Logic  Commented=on  Operator=NOT  AllPortsSameDT=off  OutDataTypeStr=boolean
  Mux3 : Mux  Inputs=2
  Overextension Torque : Fcn  Expr="- u(1)  *  (1-u(2)) * (u(2)<1) * (u(1)>0)"
  Stop Simulation1 : Stop  Commented=on
  Sum : Sum  Inputs=|+-
  overextension angle : Constant  Value=phiUpLimit
  M_stop [Nm] : Outport
  wires:
  Gain5/1 -> M_stop [Nm]/1
  Overextension Torque/1 -> Gain5/1
  Logical Operator3/1 -> Stop Simulation1/1
  Limit Ankle Range/1 -> Logical Operator3/1
  Gain2/1 -> Mux3/2
  Gain4/1 -> Gain2/1
  Sum/1 -> Gain3/1
  phi [rad]/1 -> Limit Ankle Range/1, Sum/1
  overextension angle/1 -> Sum/2
  dphi [rad/s]/1 -> Gain4/1
  Mux3/1 -> Overextension Torque/1
  Gain3/1 -> Gain1/1
  Gain1/1 -> Mux3/1

== system NeuroMuscularLibrary2/Overextension//Overflexion Joint Limit ==
  note: Overextension/Overflexion Joint Limit
  phi [rad] : Inport
  dphi [rad/s] : Inport  Port=2
  Gain1 : Gain  Gain=c_jointstop
  Gain2 : Gain  Gain=-1
  Gain3 : Gain  Gain=c_jointstop
  Gain4 : Gain  Gain=1/w_max_jointstop
  Limit Range : simulink/Logic and Bit Operations/Interval Test  Commented=on  IntervalClosedRight=on  uplimit=phi12_UpLimit + 40*pi/180  IntervalClosedLeft=on  lowlimit=phi12_LowLimit - 40*pi/180  OutDataTypeStr=boolean
  Logical Operator3 : Logic  Commented=on  Operator=NOT  AllPortsSameDT=off  OutDataTypeStr=boolean
  Mux1 : Mux  Inputs=2
  Mux3 : Mux  Inputs=2
  Overextension Torque : Fcn  Expr="- u(1)  *  (1-u(2)) * (u(2)<1) * (u(1)>0)"
  Overflexion Torque : Fcn  Expr="- u(1)  *  (1-u(2)) * (u(2)<1) * (u(1)<0)"
  Stop Simulation1 : Stop  Commented=on
  Sum : Sum  Inputs=|+-
  Sum1 : Sum  Inputs=|+-
  Sum2 : Sum
  overextension angle : Constant  Value=phiUpLimit
  overflexion angle : Constant  Value=phiLowLimit
  M_stop [Nm] : Outport
  wires:
  Mux3/1 -> Overextension Torque/1
  Gain3/1 -> Mux3/1
  dphi [rad/s]/1 -> Gain4/1
  overextension angle/1 -> Sum/2
  phi [rad]/1 -> Sum/1, Sum1/1, Limit Range/1
  Sum/1 -> Gain3/1
  Gain4/1 -> Gain2/1, Mux1/2
  Gain1/1 -> Mux1/1
  Sum1/1 -> Gain1/1
  overflexion angle/1 -> Sum1/2
  Mux1/1 -> Overflexion Torque/1
  Sum2/1 -> M_stop [Nm]/1
  Gain2/1 -> Mux3/2
  Overflexion Torque/1 -> Sum2/2
  Overextension Torque/1 -> Sum2/1
  Limit Range/1 -> Logical Operator3/1
  Logical Operator3/1 -> Stop Simulation1/1

== system NeuroMuscularLibrary2/Pos//Rot Sensor ==
  Gain2 : Gain  Gain=-1
  Mux : Mux  Inputs=3
  PS-Simulink Converter : nesl_utility/PS-Simulink Converter  PhysicalDomain=network_engine_domain  SubClassName=ps_output  LeftPortType=input  RightPortType=output  PseudoPeriodic=off  Frequencies=[]  Unit=m  AffineConversion=off
  PS-Simulink Converter1 : nesl_utility/PS-Simulink Converter  PhysicalDomain=network_engine_domain  SubClassName=ps_output  LeftPortType=input  RightPortType=output  PseudoPeriodic=off  Frequencies=[]  Unit=m  AffineConversion=off
  PS-Simulink Converter2 : nesl_utility/PS-Simulink Converter  PhysicalDomain=network_engine_domain  SubClassName=ps_output  LeftPortType=input  RightPortType=output  PseudoPeriodic=off  Frequencies=[]  Unit=m  AffineConversion=off
  PS-Simulink Converter3 : nesl_utility/PS-Simulink Converter  PhysicalDomain=network_engine_domain  SubClassName=ps_output  LeftPortType=input  RightPortType=output  PseudoPeriodic=off  Frequencies=[]  Unit=rad  AffineConversion=off
  PS-Simulink Converter4 : nesl_utility/PS-Simulink Converter  PhysicalDomain=network_engine_domain  SubClassName=ps_output  LeftPortType=input  RightPortType=output  PseudoPeriodic=off  Frequencies=[]  Unit=rad  AffineConversion=off
  Position Sensor : sm_lib/Frames and Transforms/Transform Sensor  MeasurementFrame=World  SenseAngle=on  SenseAxis=on  SenseAngle1=off  SenseAngle2=off  SenseAngle3=off  SenseQ=off  SenseR=off  SenseOmegaX=off  SenseOmegaY=off  SenseOmegaZ=off  SenseOmega1=off  SenseOmega2=off  SenseOmega3=off  SenseQDot=off  SenseRDot=off  SenseAlphaX=off  SenseAlphaY=off  SenseAlphaZ=off  SenseAlpha1=off  SenseAlpha2=off  SenseAlpha3=off  SenseQDDot=off  SenseRDDot=off  SenseX=on  SenseY=on  SenseZ=on  SenseRad=off  SenseAzim=off  SenseDist=off  SenseInc=off  SenseXDot=off  SenseYDot=off  SenseZDot=off  SenseRadDot=off  SenseAzimDot=off  SenseDistDot=off  SenseIncDot=off  SenseXDDot=off  SenseYDDot=off  SenseZDDot=off  SenseRadDDot=off  SenseAzimDDot=off  SenseDistDDot=off  SenseIncDDot=off
  Product : Product
  Selector : Selector  InputPortWidth=3  IndexOptions=Index vector (dialog)  Indices=[3]  OutputSizes=1
  Sign : Signum
  F : PMIOPort  Side=Left
  B : PMIOPort  Port=2  Side=Right
  Position : Outport
  Rotation : Outport  Port=2
  wires:
  PS-Simulink Converter1/1 -> Mux/2
  PS-Simulink Converter/1 -> Mux/1
  Mux/1 -> Position/1
  PS-Simulink Converter2/1 -> Mux/3
  PS-Simulink Converter4/1 -> Selector/1
  Selector/1 -> Sign/1
  PS-Simulink Converter3/1 -> Product/1
  Sign/1 -> Product/2
  Gain2/1 -> Rotation/1
  Product/1 -> Gain2/1
  connections:
  Position Sensor/RConn1 -- F/RConn1
  PS-Simulink Converter3/LConn1 -- Position Sensor/RConn2
  B/RConn1 -- Position Sensor/LConn1
  Position Sensor/RConn4 -- PS-Simulink Converter/LConn1
  PS-Simulink Converter1/LConn1 -- Position Sensor/RConn5
  PS-Simulink Converter2/LConn1 -- Position Sensor/RConn6
  PS-Simulink Converter4/LConn1 -- Position Sensor/RConn3

== system NeuroMuscularLibrary2/Position Sensor ==
  Mux : Mux  Inputs=3
  PS-Simulink Converter : nesl_utility/PS-Simulink Converter  PhysicalDomain=network_engine_domain  SubClassName=ps_output  LeftPortType=input  RightPortType=output  PseudoPeriodic=off  Frequencies=[]  Unit=m  AffineConversion=off
  PS-Simulink Converter1 : nesl_utility/PS-Simulink Converter  PhysicalDomain=network_engine_domain  SubClassName=ps_output  LeftPortType=input  RightPortType=output  PseudoPeriodic=off  Frequencies=[]  Unit=m  AffineConversion=off
  PS-Simulink Converter2 : nesl_utility/PS-Simulink Converter  PhysicalDomain=network_engine_domain  SubClassName=ps_output  LeftPortType=input  RightPortType=output  PseudoPeriodic=off  Frequencies=[]  Unit=m  AffineConversion=off
  Position Sensor : sm_lib/Frames and Transforms/Transform Sensor  MeasurementFrame=World  SenseAngle=off  SenseAxis=off  SenseAngle1=off  SenseAngle2=off  SenseAngle3=off  SenseQ=off  SenseR=off  SenseOmegaX=off  SenseOmegaY=off  SenseOmegaZ=off  SenseOmega1=off  SenseOmega2=off  SenseOmega3=off  SenseQDot=off  SenseRDot=off  SenseAlphaX=off  SenseAlphaY=off  SenseAlphaZ=off  SenseAlpha1=off  SenseAlpha2=off  SenseAlpha3=off  SenseQDDot=off  SenseRDDot=off  SenseX=on  SenseY=on  SenseZ=on  SenseRad=off  SenseAzim=off  SenseDist=off  SenseInc=off  SenseXDot=off  SenseYDot=off  SenseZDot=off  SenseRadDot=off  SenseAzimDot=off  SenseDistDot=off  SenseIncDot=off  SenseXDDot=off  SenseYDDot=off  SenseZDDot=off  SenseRadDDot=off  SenseAzimDDot=off  SenseDistDDot=off  SenseIncDDot=off
  World Frame : sm_lib/Frames and Transforms/World Frame
  Frame : PMIOPort  Side=Left
  Position : Outport
  wires:
  PS-Simulink Converter2/1 -> Mux/3
  Mux/1 -> Position/1
  PS-Simulink Converter/1 -> Mux/1
  PS-Simulink Converter1/1 -> Mux/2
  connections:
  PS-Simulink Converter2/LConn1 -- Position Sensor/RConn4
  PS-Simulink Converter/LConn1 -- Position Sensor/RConn2
  Position Sensor/RConn1 -- Frame/RConn1
  PS-Simulink Converter1/LConn1 -- Position Sensor/RConn3
  Position Sensor/LConn1 -- World Frame/RConn1
